simulink model "BloquesP1"  (R2017b)
settings: Solver=VariableStepAuto  StartTime=0.0  StopTime=5000  RelTol=1e-3
values from neighbouring files (symbols this model uses):
  A = [-s2-s3, s3, 0; s4, -s4-s5, s5; 0, s6, -s6]    [Modelación-Manjar.m]    (also in codigoP1.m)
  B = [s1; 0; 0]    [Modelación-Manjar.m]    (also in codigoP1.m)
  D = [T_a*s2;0;0]    [Modelación-Manjar.m]    (also in codigoP1.m)
  x0 = [298.15,298.15,298.15]    [Modelación-Manjar.m]    (also in codigoP1.m)
settings Model: Creator=Pia  LastModifiedBy=Pia

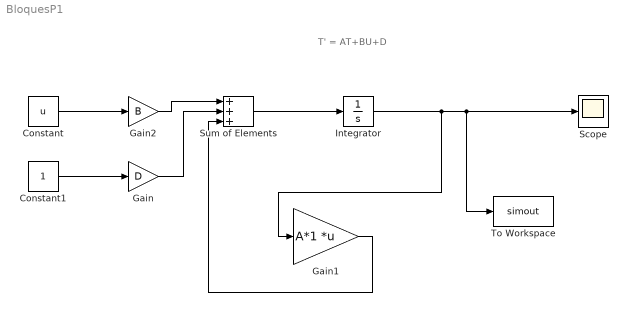
== system BloquesP1 ==
  note: T' = AT+BU+D
  Constant : Constant  Value=u
  Constant1 : Constant
  Gain : Gain  Gain=D
  Gain1 : Gain  Gain=A*1  Multiplication=Matrix(K*u) (u vector)
  Gain2 : Gain  Gain=B
  Integrator : Integrator  InitialCondition=x0
  Scope : Scope
  Sum of Elements : Sum  Inputs=+++
  To Workspace : ToWorkspace  VariableName=simout  SampleTime=-1
  wires:
  Integrator/1 -> Gain1/1, To Workspace/1, Scope/1
  Gain1/1 -> Sum of Elements/3
  Gain/1 -> Sum of Elements/2
  Gain2/1 -> Sum of Elements/1
  Sum of Elements/1 -> Integrator/1
  Constant/1 -> Gain2/1
  Constant1/1 -> Gain/1
